simulink model "Versuch_1_Aufgabe_1"  (R2023b)
settings: Solver=VariableStepAuto  StartTime=0.0  StopTime=10.0  RelTol=1e-3
values from neighbouring files (symbols this model uses):
  AB = 0.0226    [Versuch_1_Aufgabe_1_Skript.m]
  h = 0.1    [Versuch_1_Aufgabe_1_Skript.m]
  KR = KR_array(count)    [Versuch_1_Aufgabe_1_Skript.m]
  sim_time = 70    [Versuch_1_Aufgabe_1_Skript.m]
settings Model: Creator=danie  LastModifiedBy=danie

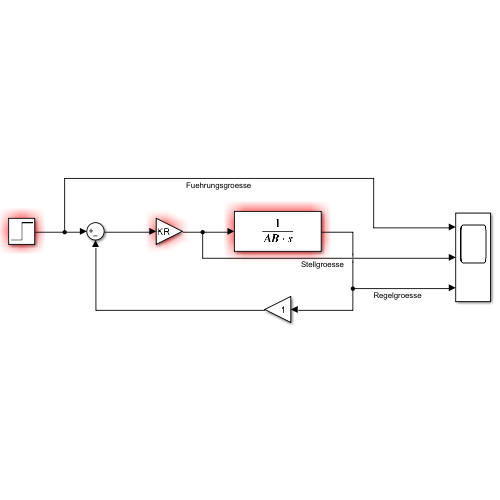
[thumbnail: Simulink's stored preview of the top-level diagram]
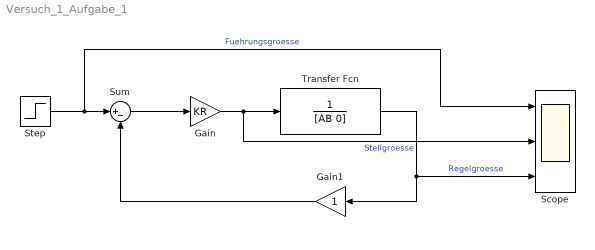
== system Versuch_1_Aufgabe_1 ==
  Gain : Gain  Gain=KR
  Gain1 : Gain
  Scope : Scope  NumInputPorts=3
  Step : Step  Time=sim_time  Before=h  SampleTime=0
  Sum : Sum  Inputs=|+-
  Transfer Fcn : TransferFcn  Denominator=[AB 0]
  wires:
  Gain/1 -> Scope/2, Transfer Fcn/1  "Stellgroesse"
  Sum/1 -> Gain/1
  Gain1/1 -> Sum/2
  Transfer Fcn/1 -> Scope/3, Gain1/1  "Regelgroesse"
  Step/1 -> Scope/1, Sum/1  "Fuehrungsgroesse"
